simulink model "control_system_obsmin"  (R2020a)
settings: Solver=VariableStepAuto  StartTime=0.0  StopTime=1000  RelTol=1e-3
InitFcn:
  | LAB2
values from neighbouring files (symbols this model uses):
  A = [-0.342 0 0.0318; 0 -0.0716 0.0318; 0.0204 0.0204 -0.0423]    [LAB2.m]
  B = [0.159 0; 0 0.159; 0 0]    [LAB2.m]
  F = A20-L_min*A10    [LAB2.m]
  G = (A20-L_min*A10)*L_min + (A2m-L_min*A1m)    [LAB2.m]
  H = B0-L_min*Bm    [LAB2.m]
  K = K_(:,1:3)    [LAB2.m]
  L_min = place(A20',A10',-Wn0)'    [LAB2.m]
  N = K_(:,4:end)    [LAB2.m]
settings Model: Creator=paulogil  LastModifiedBy=joaom
settings OptimizationCC: LifeSpan=inf
settings DebuggingCC: SFExecutionAtInitializationDiag=none  ArithmeticOperatorsInVariantConditions=warning
settings SFSimCC: CustomCodeUndefinedFunction=UseInterfaceOnly
settings CodeAppCC: StateflowObjectComments=on

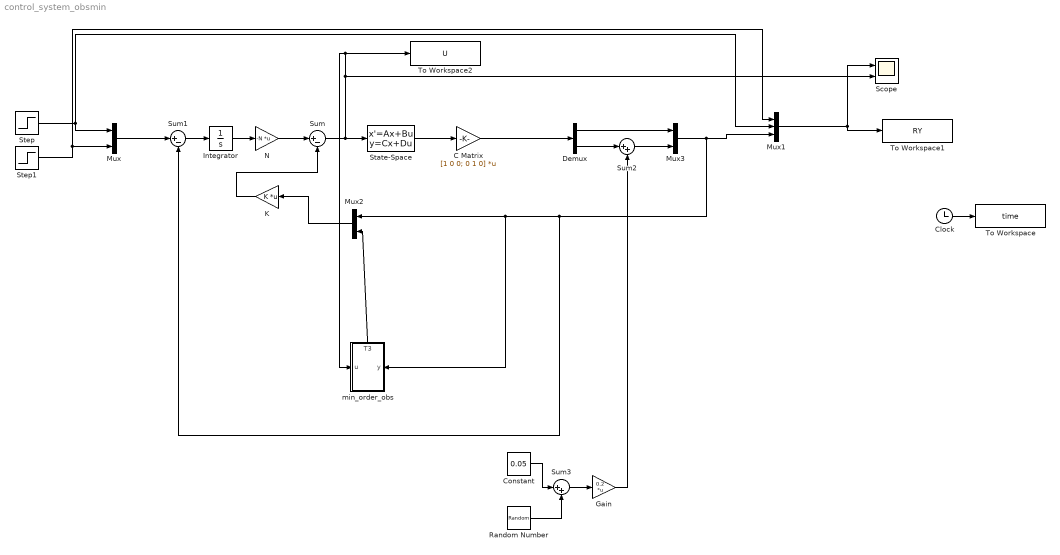
== system control_system_obsmin ==
  C Matrix : Gain  Gain=[1 0 0; 0 1 0]  Multiplication=Matrix(K*u)
  Clock : Clock
  Constant : Constant  Value=0.05
  Demux : Demux  Outputs=2
  Gain : Gain  Gain=0.2  Multiplication=Matrix(K*u)
  Integrator : Integrator
  K : Gain  Gain=K  Multiplication=Matrix(K*u)
  Mux : Mux  Inputs=2
  Mux1 : Mux  Inputs=3
  Mux2 : Mux  Inputs=2
  Mux3 : Mux  Inputs=2
  N : Gain  Gain=-N  Multiplication=Matrix(K*u)
  Random Number : RandomNumber  Variance=0.001  SampleTime=0.1
  Scope : Scope  NumInputPorts=2
  State-Space : StateSpace  A=A  B=B  C=eye(3)  D=zeros(3,2)  InitialCondition=0
  Step : Step  Time=0  After=0.5  SampleTime=0
  Step1 : Step  After=0.7  SampleTime=0
  Sum : Sum  Inputs=|+-
  Sum1 : Sum  Inputs=|+-
  Sum2 : Sum  Inputs=|++
  Sum3 : Sum  Inputs=|++
  To Workspace : ToWorkspace  VariableName=time  SaveFormat=Timeseries  SampleTime=-1
  To Workspace1 : ToWorkspace  VariableName=RY  SaveFormat=Timeseries  SampleTime=-1
  To Workspace2 : ToWorkspace  VariableName=U  SaveFormat=Timeseries  SampleTime=-1
  min_order_obs : Subsystem
      settings: PortSchema="{\"entries\":[{\"content\":{\"sides\":[{\"content\":{\"connectorIds\":[\"In1\"]},\"type\":\"ConnectorPlacement.EquallySpacedRectSide\",\"uuid\":\"c7da1c28-c8df-40b7-86e4-25906281d971\"},{\"content\":{\"connectorIds\":[\"In2\"],\"side\":\"RIGHT\"},\"type\":\"ConnectorPlacement.EquallySpacedRectSide\",\"uuid\":\"dfcd5ef7-36f8-48c2-a26a-9576f1f2beae\"},{\"content\":{\"connectorIds\":[\"Out1\"],\"side\":\"TOP\"},\"type\":\"ConnectorPlacement.EquallySpacedRectSide\",\"uuid\":\"aacb2fb5-39b3-406f-b761-71602a16b32b\"}]},\"type\":\"ConnectorPlacement.EquallySpacedConnector\",\"uuid\":\"facd32b2-a411-488b-bac6-8ba9c6a22f57\"}],\"packageUris\":[\"http://schema.mathworks.com/mf0/Connector/19700101\"],\"version\":\"1.0\"}"
  wires:
  State-Space/1 -> C Matrix/1
  Sum/1 -> min_order_obs/1(u), To Workspace2/1, Scope/2, State-Space/1
  N/1 -> Sum/1
  Mux1/1 -> To Workspace1/1, Scope/1
  Clock/1 -> To Workspace/1
  Integrator/1 -> N/1
  Sum1/1 -> Integrator/1
  C Matrix/1 -> Demux/1
  Step/1 -> Mux1/2, Mux/1
  Step1/1 -> Mux1/1, Mux/2
  Mux/1 -> Sum1/1
  min_order_obs/1(T3) -> Mux2/2
  Mux2/1 -> K/1
  K/1 -> Sum/2
  Constant/1 -> Sum3/1
  Sum3/1 -> Gain/1
  Random Number/1 -> Sum3/2
  Gain/1 -> Sum2/2
  Demux/1 -> Mux3/1
  Demux/2 -> Sum2/1
  Sum2/1 -> Mux3/2
  Mux3/1 -> Sum1/2, min_order_obs/2(y), Mux2/1, Mux1/3

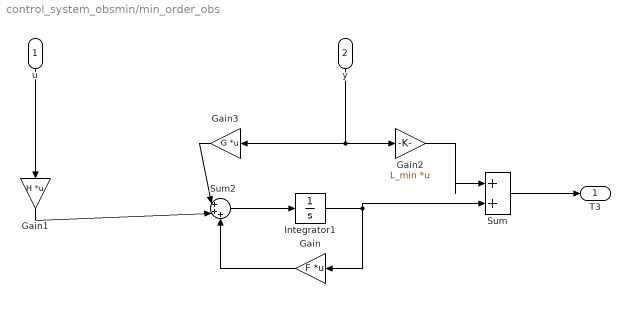
== system control_system_obsmin/min_order_obs ==
  u : Inport
  y : Inport  Port=2
  Gain : Gain  Gain=F  Multiplication=Matrix(K*u)
  Gain1 : Gain  Gain=H  Multiplication=Matrix(K*u)
  Gain2 : Gain  Gain=L_min  Multiplication=Matrix(K*u)
  Gain3 : Gain  Gain=G  Multiplication=Matrix(K*u)
  Integrator1 : Integrator
  Sum : Sum  Inputs=|++
  Sum2 : Sum  Inputs=|+++
  T3 : Outport
  wires:
  Sum2/1 -> Integrator1/1
  Gain/1 -> Sum2/3
  Integrator1/1 -> Gain/1, Sum/2
  u/1 -> Gain1/1
  Gain1/1 -> Sum2/2
  Gain2/1 -> Sum/1
  y/1 -> Gain3/1, Gain2/1
  Gain3/1 -> Sum2/1
  Sum/1 -> T3/1
